simulink model "Sistema_in_catena_chiusa"  (R2014a)
settings: Solver=ode45  StartTime=0.0  StopTime=20  RelTol=1e-3
undefined symbols (not defined in the file or in its folder): Kc
libraries: cstblocks x2
settings Model: Creator=Davide  LastModifiedBy=Davide
settings DataIOCC: LimitDataPoints=off  SignalLoggingSaveFormat=ModelDataLogs

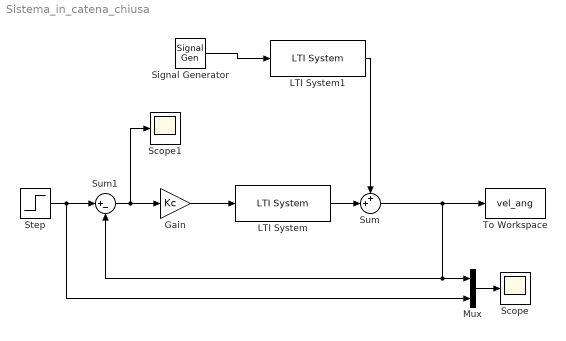
== system Sistema_in_catena_chiusa ==
  Gain : Gain  Gain=Kc
  LTI System : cstblocks/LTI System  sys=F1  IC=[]
  LTI System1 : cstblocks/LTI System  sys=F2  IC=[]
  Mux : Mux  Inputs=2
  Scope : Scope
  Scope1 : Scope
  Signal Generator : SignalGenerator  WaveForm=square  Amplitude=0.05  Frequency=0.1
  Step : Step  Time=0  SampleTime=0
  Sum : Sum  Inputs=++|
  Sum1 : Sum  Inputs=|+-
  To Workspace : ToWorkspace  VariableName=vel_ang  SampleTime=-1
  wires:
  Step/1 -> Sum1/1, Mux/2
  LTI System/1 -> Sum/2
  LTI System1/1 -> Sum/1
  Signal Generator/1 -> LTI System1/1
  Sum/1 -> To Workspace/1, Sum1/2, Mux/1
  Mux/1 -> Scope/1
  Sum1/1 -> Gain/1, Scope1/1
  Gain/1 -> LTI System/1
